simulink model "sampleModel15090_1"  (R2023b)
settings: Solver=VariableStepAuto  StartTime=0.0  StopTime=10.0  RelTol=1e-3
libraries: hdlsllib x12, simulink x2
settings Model: Creator=Tsmc  LastModifiedBy=Tsmc

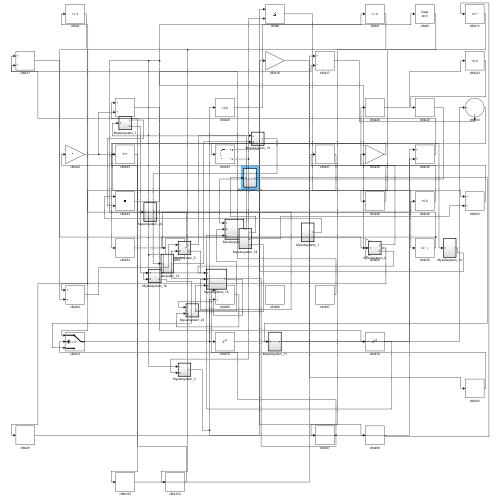
[thumbnail: Simulink's stored preview of the top-level diagram]
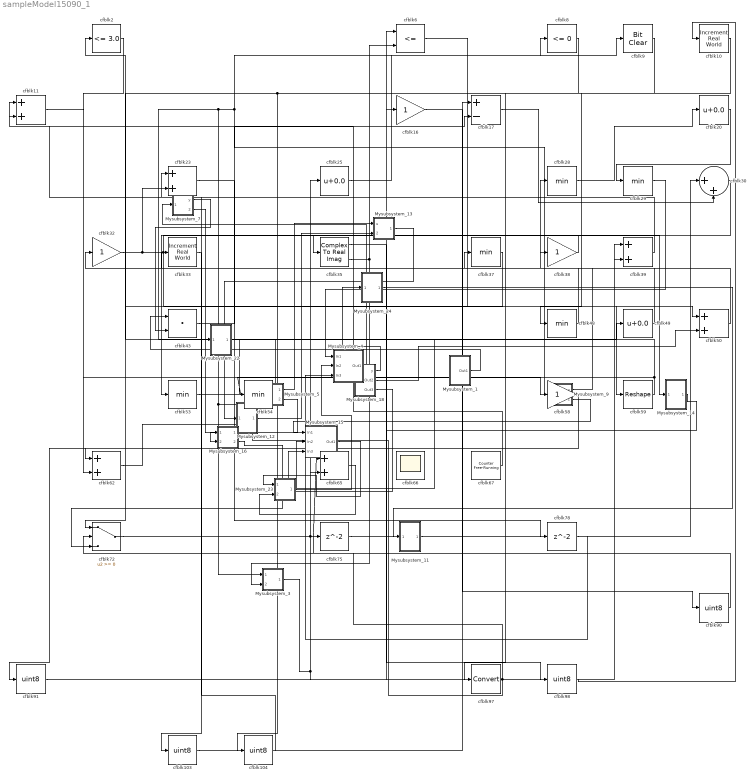
== system sampleModel15090_1 ==
  Mysubsystem_1 : Subsystem  TreatAsAtomicUnit=on  RTWFcnName=Mysubsystem_1
      settings: RTWFcnNameOpts=User specified  RTWFileNameOpts=Use function name
  Mysubsystem_11 : Subsystem  TreatAsAtomicUnit=on  RTWFcnName=Mysubsystem_11
      settings: RTWFcnNameOpts=User specified  RTWFileNameOpts=Use function name
  Mysubsystem_12 : Subsystem  TreatAsAtomicUnit=on  RTWFcnName=Mysubsystem_12
      settings: RTWFcnNameOpts=User specified  RTWFileNameOpts=Use function name
  Mysubsystem_13 : Subsystem  TreatAsAtomicUnit=on  RTWFcnName=Mysubsystem_13
      settings: RTWFcnNameOpts=User specified  RTWFileNameOpts=Use function name
  Mysubsystem_14 : Subsystem  TreatAsAtomicUnit=on  RTWFcnName=Mysubsystem_14
      settings: RTWFcnNameOpts=User specified  RTWFileNameOpts=Use function name
  Mysubsystem_15 : Subsystem  TreatAsAtomicUnit=on  RTWFcnName=Mysubsystem_15
      settings: RTWFcnNameOpts=User specified  RTWFileNameOpts=Use function name
  Mysubsystem_16 : Subsystem  TreatAsAtomicUnit=on  RTWFcnName=Mysubsystem_16
      settings: RTWFcnNameOpts=User specified  RTWFileNameOpts=Use function name
  Mysubsystem_18 : Subsystem  TreatAsAtomicUnit=on  RTWFcnName=Mysubsystem_18
      settings: RTWFcnNameOpts=User specified  RTWFileNameOpts=Use function name
  Mysubsystem_22 : Subsystem  TreatAsAtomicUnit=on  RTWFcnName=Mysubsystem_22
      settings: RTWFcnNameOpts=User specified  RTWFileNameOpts=Use function name
  Mysubsystem_23 : Subsystem  TreatAsAtomicUnit=on  RTWFcnName=Mysubsystem_23
      settings: RTWFcnNameOpts=User specified  RTWFileNameOpts=Use function name
  Mysubsystem_24 : Subsystem  TreatAsAtomicUnit=on  RTWFcnName=Mysubsystem_24
      settings: RTWFcnNameOpts=User specified  RTWFileNameOpts=Use function name
  Mysubsystem_3 : Subsystem  TreatAsAtomicUnit=on  RTWFcnName=Mysubsystem_3
      settings: RTWFcnNameOpts=User specified  RTWFileNameOpts=Use function name
  Mysubsystem_4 : Subsystem  TreatAsAtomicUnit=on  RTWFcnName=Mysubsystem_4
      settings: RTWFcnNameOpts=User specified  RTWFileNameOpts=Use function name
  Mysubsystem_5 : Subsystem  TreatAsAtomicUnit=on  RTWFcnName=Mysubsystem_5
      settings: RTWFcnNameOpts=User specified  RTWFileNameOpts=Use function name
  Mysubsystem_7 : Subsystem  TreatAsAtomicUnit=on  RTWFcnName=Mysubsystem_7
      settings: RTWFcnNameOpts=User specified  RTWFileNameOpts=Use function name
  Mysubsystem_9 : Subsystem  TreatAsAtomicUnit=on  RTWFcnName=Mysubsystem_9
      settings: RTWFcnNameOpts=User specified  RTWFileNameOpts=Use function name
  cfblk10 : hdlsllib/Math Operations/Increment Real World
  cfblk{90..91,98,103..104} (5 alike) : DataTypeConversion  OutDataTypeStr=uint8  SaturateOnIntegerOverflow=off  RndMeth=Floor
  cfblk{11,23,39,50,62,65} (6 alike) : Sum
  cfblk{16,32,38,58} (4 alike) : Gain
  cfblk17 : Sum  Inputs=+-
  cfblk2 : hdlsllib/Logic and Bit Operations/Compare To Constant  relop=<=  const=3.0  OutDataTypeStr=boolean
  cfblk20 : Bias  Bias=0.0  SaturateOnIntegerOverflow=off
  cfblk25 : Bias  Bias=0.0  SaturateOnIntegerOverflow=off
  cfblk{28..29,37,48,53..54} (6 alike) : MinMax
  cfblk30 : Sum  Inputs=|++
  cfblk33 : hdlsllib/Math Operations/Increment Real World
  cfblk35 : ComplexToRealImag
  cfblk43 : DotProduct  OutDataTypeStr=Inherit: Inherit via internal rule
  cfblk49 : Bias  Bias=0.0  SaturateOnIntegerOverflow=off
  cfblk59 : Reshape
  cfblk6 : RelationalOperator  Operator=<=  OutDataTypeStr=boolean  InputSameDT=off
  cfblk66 : Scope
      settings: Floating=on
  cfblk67 : hdlsllib/Sources/Counter Free-Running  NumBits=16  tsamp=-1
  cfblk72 : Switch  SaturateOnIntegerOverflow=off  InputSameDT=off
  cfblk75 : Delay  SampleTime=1
  cfblk78 : Delay  SampleTime=1
  cfblk8 : hdlsllib/Logic and Bit Operations/Compare To Zero  relop=<=  OutDataTypeStr=boolean
  cfblk9 : simulink/Logic and Bit Operations/Bit Clear  iBit=0
      settings: LibrarySourceBlock=|
      | hdlsllib/Logic and Bit
      | Operations/Bit Clear
  cfblk97 : DataTypeConversion  SaturateOnIntegerOverflow=off  RndMeth=Floor
  wires:
  cfblk32/1 -> Mysubsystem_14/1(In1), cfblk50/1, cfblk23/2
  cfblk72/1 -> cfblk25/1, cfblk65/1
  cfblk6/1 -> cfblk59/1
  cfblk35/2 -> Mysubsystem_3/2(In2), cfblk6/2
  cfblk20/1 -> cfblk29/1
  cfblk25/1 -> cfblk8/1
  cfblk48/1 -> cfblk2/1
  cfblk67/1 -> cfblk11/1
  cfblk28/1 -> cfblk20/1
  cfblk30/1 -> cfblk53/1
  cfblk50/1 -> cfblk28/1
  cfblk8/1 -> cfblk62/1, cfblk104/1
  cfblk10/1 -> cfblk97/1
  cfblk2/1 -> cfblk62/2
  cfblk43/1 -> cfblk17/2
  cfblk17/1 -> cfblk30/2
  cfblk53/1 -> cfblk49/1
  cfblk37/1 -> cfblk72/1
  cfblk9/1 -> cfblk48/1
  cfblk38/1 -> cfblk35/1
  cfblk49/1 -> cfblk38/1
  cfblk59/1 -> cfblk54/1, cfblk32/1
  cfblk11/1 -> cfblk58/1
  cfblk54/1 -> cfblk23/1
  cfblk39/1 -> cfblk11/2
  cfblk75/1 -> cfblk30/1
  cfblk23/1 -> cfblk78/1
  cfblk78/1 -> cfblk39/1
  cfblk16/1 -> cfblk90/1
  cfblk90/1 -> cfblk72/2
  cfblk58/1 -> cfblk91/1
  cfblk91/1 -> cfblk16/1
  cfblk97/1 -> Mysubsystem_5/2(In2), cfblk75/1
  cfblk35/1 -> cfblk98/1
  cfblk98/1 -> cfblk10/1
  cfblk33/1 -> cfblk103/1
  cfblk103/1 -> cfblk17/1
  cfblk104/1 -> cfblk33/1
  Mysubsystem_1/1(Out1) -> cfblk43/1
  Mysubsystem_3/1(Out1) -> cfblk39/2, cfblk65/2
  cfblk29/1 -> Mysubsystem_4/1(In1)
  cfblk62/1 -> Mysubsystem_5/1(In1)
  Mysubsystem_4/1(Out1) -> Mysubsystem_7/1(In1)
  Mysubsystem_7/1(y) -> cfblk43/2
  Mysubsystem_9/1(y) -> cfblk37/1
  Mysubsystem_11/1(Out1) -> Mysubsystem_4/3(In3)
  Mysubsystem_5/1(Out1) -> Mysubsystem_13/1(u)
  Mysubsystem_12/1(Out1) -> Mysubsystem_13/2(In2)
  Mysubsystem_13/1(Out1) -> Mysubsystem_12/1(In1)
  Mysubsystem_14/1(Out1) -> cfblk6/1
  Mysubsystem_9/2(Out2) -> Mysubsystem_15/1(In1)
  Mysubsystem_16/1(Out1) -> Mysubsystem_9/1(In1), cfblk9/1, Mysubsystem_22/1(In1), Mysubsystem_3/1(In1)
  Mysubsystem_7/2(Out2) -> Mysubsystem_16/1(In1)
  Mysubsystem_5/2(Out2) -> Mysubsystem_16/2(In2)
  Mysubsystem_16/2(Out2) -> cfblk72/3
  Mysubsystem_18/2(Out2) -> cfblk50/2
  Mysubsystem_18/3(Out3) -> Mysubsystem_15/3(In3)
  Mysubsystem_22/1(Out1) -> Mysubsystem_15/2(In2)
  Mysubsystem_15/1(Out1) -> Mysubsystem_23/1(In1)
  cfblk65/1 -> Mysubsystem_23/2(In2)
  Mysubsystem_23/1(Out1) -> Mysubsystem_4/2(In2)
  Mysubsystem_18/1(y) -> Mysubsystem_24/1(In1)
  Mysubsystem_24/1(Out1) -> Mysubsystem_11/1(In1)

== system sampleModel15090_1/Mysubsystem_1 ==
  cfblk34 : hdlsllib/Math Operations/Increment Real World
  cfblk46 : Abs  SaturateOnIntegerOverflow=off
  cfblk80 : Delay  SampleTime=1
  Out1 : Outport
  wires:
  cfblk46/1 -> Out1/1, cfblk80/1
  cfblk34/1 -> cfblk46/1
  cfblk80/1 -> cfblk34/1

== system sampleModel15090_1/Mysubsystem_11 ==
  In1 : Inport
  cfblk51 : Reshape
  cfblk88 : DataTypeConversion  OutDataTypeStr=uint8  SaturateOnIntegerOverflow=off  RndMeth=Floor
  cfblk89 : DataTypeConversion  OutDataTypeStr=uint8  SaturateOnIntegerOverflow=off  RndMeth=Floor
  Out1 : Outport
  wires:
  cfblk88/1 -> Out1/1
  cfblk51/1 -> cfblk88/1
  cfblk89/1 -> cfblk51/1
  In1/1 -> cfblk89/1

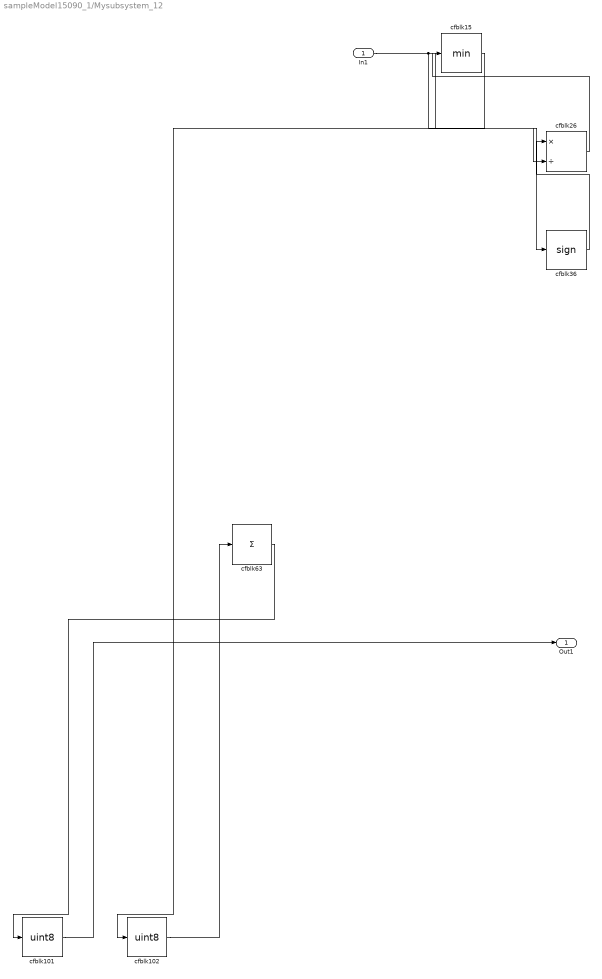
== system sampleModel15090_1/Mysubsystem_12 ==
  In1 : Inport
  cfblk101 : DataTypeConversion  OutDataTypeStr=uint8  SaturateOnIntegerOverflow=off  RndMeth=Floor
  cfblk102 : DataTypeConversion  OutDataTypeStr=uint8  SaturateOnIntegerOverflow=off  RndMeth=Floor
  cfblk15 : MinMax
  cfblk26 : Product  Inputs=*/  RndMeth=Zero  SaturateOnIntegerOverflow=on
  cfblk36 : Signum
  cfblk63 : Sum  Inputs=+
  Out1 : Outport
  wires:
  cfblk36/1 -> cfblk26/1
  cfblk101/1 -> Out1/1
  cfblk26/1 -> cfblk15/1
  In1/1 -> cfblk36/1, cfblk26/2
  cfblk63/1 -> cfblk101/1
  cfblk102/1 -> cfblk63/1
  cfblk15/1 -> cfblk102/1

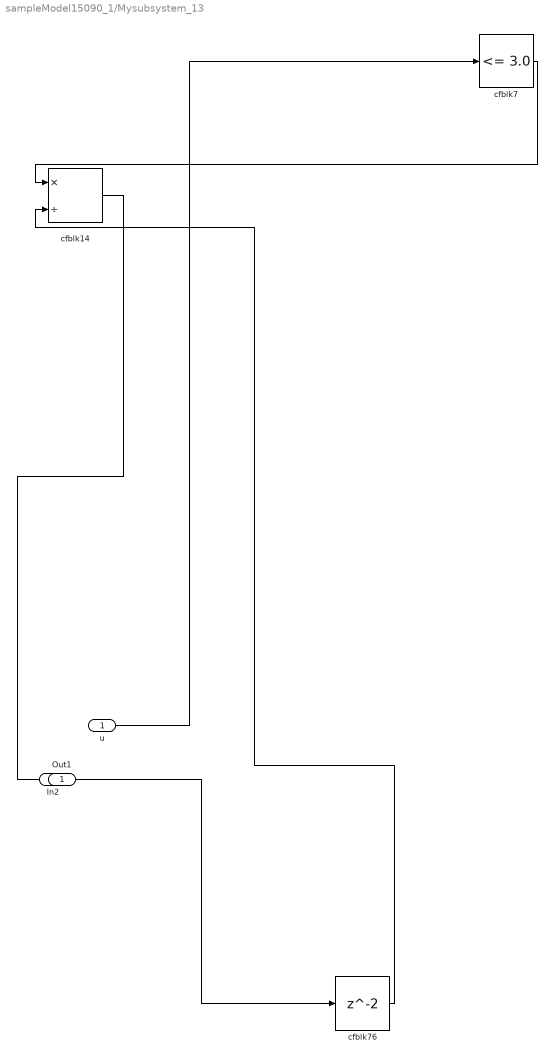
== system sampleModel15090_1/Mysubsystem_13 ==
  u : Inport
  In2 : Inport  Port=2
  cfblk14 : Product  Inputs=*/  RndMeth=Zero  SaturateOnIntegerOverflow=on
  cfblk7 : hdlsllib/Logic and Bit Operations/Compare To Constant  relop=<=  const=3.0  OutDataTypeStr=boolean
  cfblk76 : Delay  SampleTime=1
  Out1 : Outport
  wires:
  cfblk7/1 -> cfblk14/1
  In2/1 -> cfblk76/1
  cfblk14/1 -> Out1/1
  cfblk76/1 -> cfblk14/2
  u/1 -> cfblk7/1

== system sampleModel15090_1/Mysubsystem_14 ==
  In1 : Inport
  cfblk40 : Abs  SaturateOnIntegerOverflow=off
  cfblk79 : Delay  SampleTime=1
  Out1 : Outport
  wires:
  cfblk40/1 -> cfblk79/1
  In1/1 -> cfblk40/1
  cfblk79/1 -> Out1/1

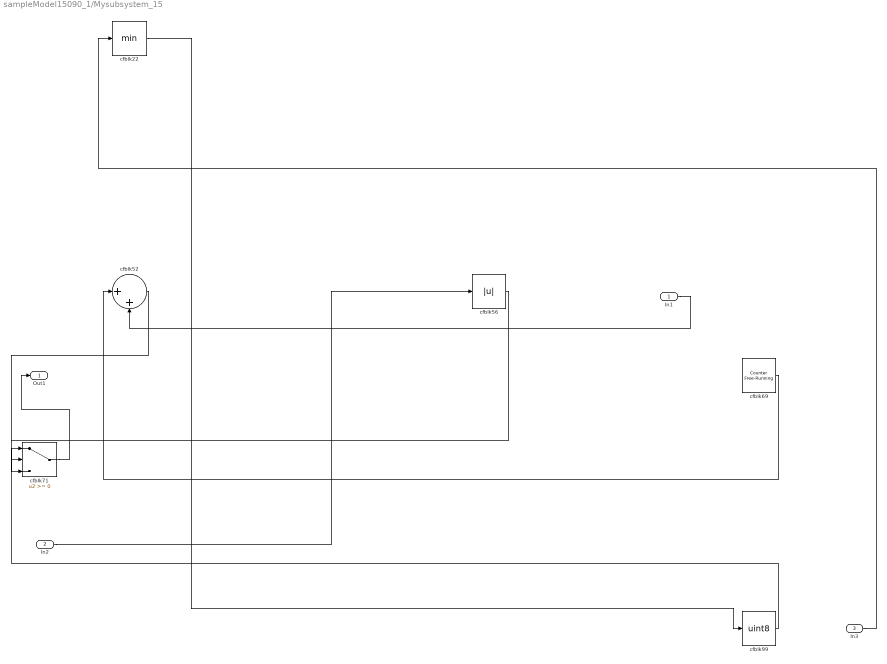
== system sampleModel15090_1/Mysubsystem_15 ==
  In1 : Inport
  In2 : Inport  Port=2
  In3 : Inport  Port=3
  cfblk22 : MinMax
  cfblk52 : Sum  Inputs=|++
  cfblk56 : Abs  SaturateOnIntegerOverflow=off
  cfblk69 : hdlsllib/Sources/Counter Free-Running  NumBits=16  tsamp=-1
  cfblk71 : Switch  SaturateOnIntegerOverflow=off  InputSameDT=off
  cfblk99 : DataTypeConversion  OutDataTypeStr=uint8  SaturateOnIntegerOverflow=off  RndMeth=Floor
  Out1 : Outport
  wires:
  cfblk69/1 -> cfblk52/1
  cfblk52/1 -> cfblk71/2
  cfblk22/1 -> cfblk99/1
  cfblk99/1 -> cfblk71/1
  cfblk56/1 -> cfblk71/3
  cfblk71/1 -> Out1/1
  In2/1 -> cfblk56/1
  In3/1 -> cfblk22/1
  In1/1 -> cfblk52/2

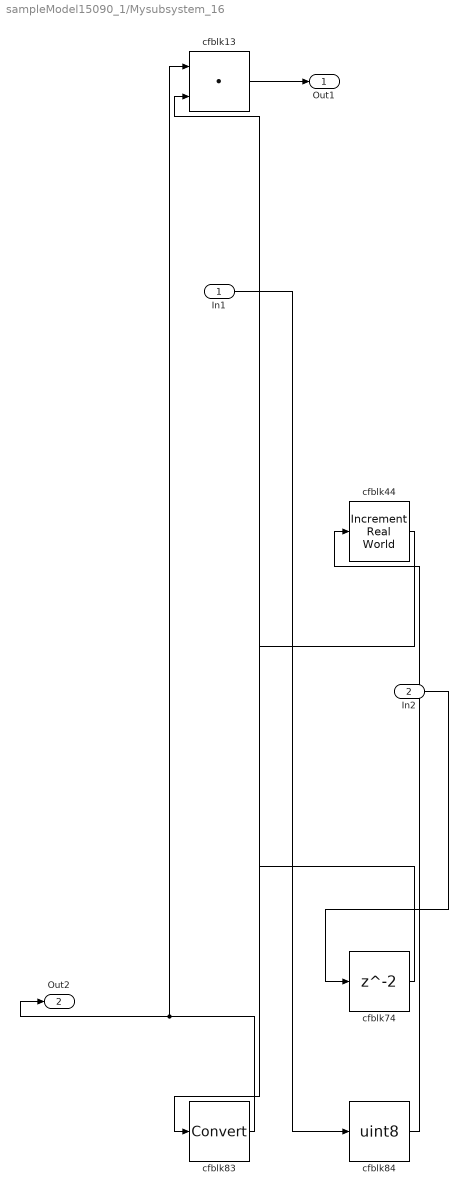
== system sampleModel15090_1/Mysubsystem_16 ==
  In1 : Inport
  In2 : Inport  Port=2
  cfblk13 : DotProduct  OutDataTypeStr=Inherit: Inherit via internal rule
  cfblk44 : hdlsllib/Math Operations/Increment Real World
  cfblk74 : Delay  SampleTime=1
  cfblk83 : DataTypeConversion  SaturateOnIntegerOverflow=off  RndMeth=Floor
  cfblk84 : DataTypeConversion  OutDataTypeStr=uint8  SaturateOnIntegerOverflow=off  RndMeth=Floor
  Out1 : Outport
  Out2 : Outport  Port=2
  wires:
  cfblk44/1 -> cfblk83/1
  cfblk84/1 -> cfblk44/1
  In2/1 -> cfblk74/1
  cfblk13/1 -> Out1/1
  cfblk74/1 -> cfblk13/2
  cfblk83/1 -> Out2/1, cfblk13/1
  In1/1 -> cfblk84/1

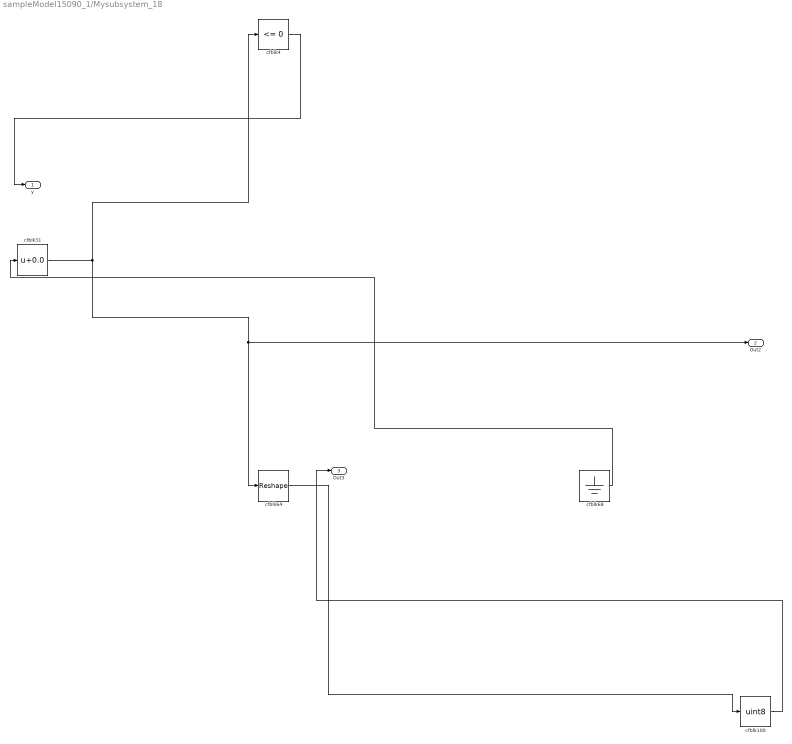
== system sampleModel15090_1/Mysubsystem_18 ==
  cfblk100 : DataTypeConversion  OutDataTypeStr=uint8  SaturateOnIntegerOverflow=off  RndMeth=Floor
  cfblk31 : Bias  Bias=0.0  SaturateOnIntegerOverflow=off
  cfblk4 : hdlsllib/Logic and Bit Operations/Compare To Zero  relop=<=  OutDataTypeStr=boolean
  cfblk64 : Reshape
  cfblk68 : Ground
  y : Outport
  Out2 : Outport  Port=2
  Out3 : Outport  Port=3
  wires:
  cfblk31/1 -> Out2/1, cfblk64/1, cfblk4/1
  cfblk64/1 -> cfblk100/1
  cfblk68/1 -> cfblk31/1
  cfblk4/1 -> y/1
  cfblk100/1 -> Out3/1

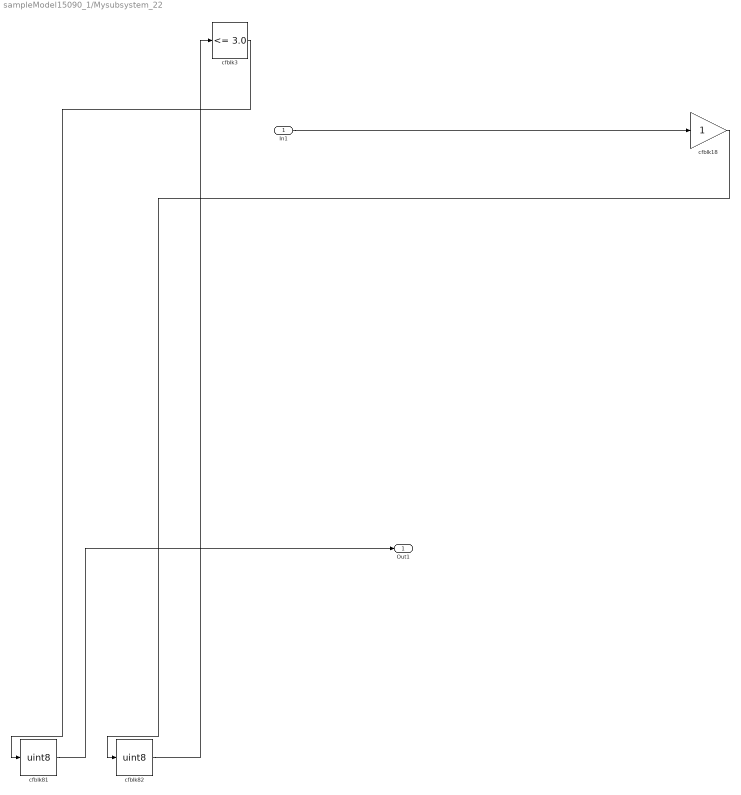
== system sampleModel15090_1/Mysubsystem_22 ==
  In1 : Inport
  cfblk18 : Gain
  cfblk3 : hdlsllib/Logic and Bit Operations/Compare To Constant  relop=<=  const=3.0  OutDataTypeStr=boolean
  cfblk81 : DataTypeConversion  OutDataTypeStr=uint8  SaturateOnIntegerOverflow=off  RndMeth=Floor
  cfblk82 : DataTypeConversion  OutDataTypeStr=uint8  SaturateOnIntegerOverflow=off  RndMeth=Floor
  Out1 : Outport
  wires:
  cfblk18/1 -> cfblk82/1
  In1/1 -> cfblk18/1
  cfblk82/1 -> cfblk3/1
  cfblk3/1 -> cfblk81/1
  cfblk81/1 -> Out1/1

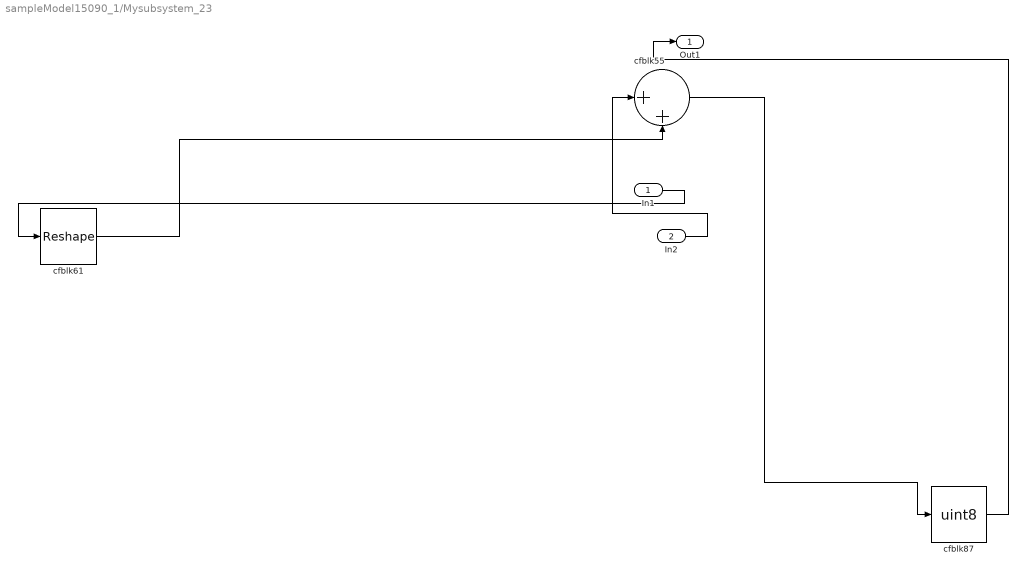
== system sampleModel15090_1/Mysubsystem_23 ==
  In1 : Inport
  In2 : Inport  Port=2
  cfblk55 : Sum  Inputs=|++
  cfblk61 : Reshape
  cfblk87 : DataTypeConversion  OutDataTypeStr=uint8  SaturateOnIntegerOverflow=off  RndMeth=Floor
  Out1 : Outport
  wires:
  cfblk55/1 -> cfblk87/1
  cfblk61/1 -> cfblk55/2
  In2/1 -> cfblk55/1
  In1/1 -> cfblk61/1
  cfblk87/1 -> Out1/1

== system sampleModel15090_1/Mysubsystem_24 ==
  In1 : Inport
  cfblk21 : Signum
  cfblk60 : Reshape
  Out1 : Outport
  wires:
  cfblk21/1 -> cfblk60/1
  In1/1 -> cfblk21/1
  cfblk60/1 -> Out1/1

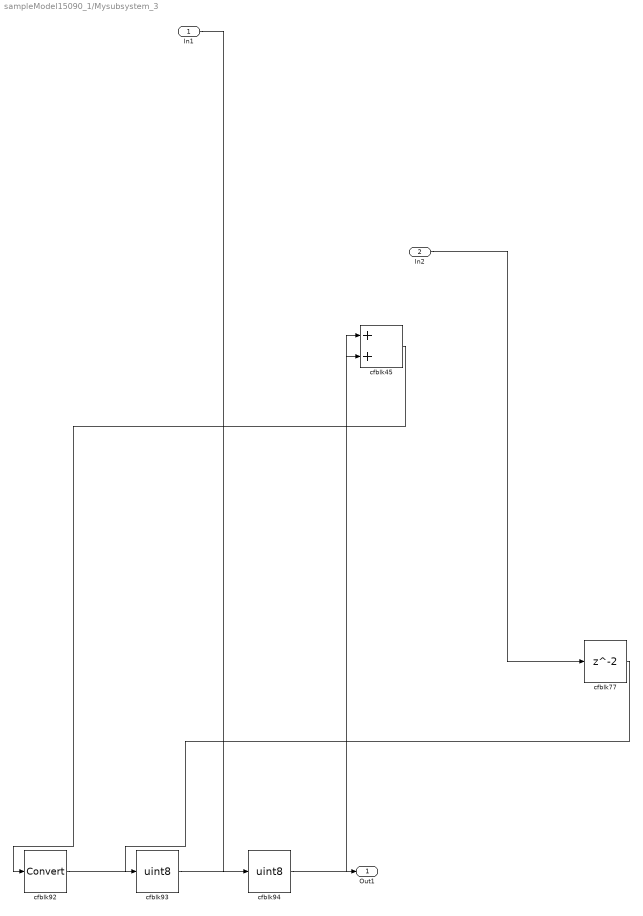
== system sampleModel15090_1/Mysubsystem_3 ==
  In1 : Inport
  In2 : Inport  Port=2
  cfblk45 : Sum
  cfblk77 : Delay  SampleTime=1
  cfblk92 : DataTypeConversion  SaturateOnIntegerOverflow=off  RndMeth=Floor
  cfblk93 : DataTypeConversion  OutDataTypeStr=uint8  SaturateOnIntegerOverflow=off  RndMeth=Floor
  cfblk94 : DataTypeConversion  OutDataTypeStr=uint8  SaturateOnIntegerOverflow=off  RndMeth=Floor
  Out1 : Outport
  wires:
  In2/1 -> cfblk77/1
  cfblk45/1 -> cfblk92/1
  cfblk92/1 -> Out1/1
  In1/1 -> cfblk94/1
  cfblk77/1 -> cfblk93/1
  cfblk94/1 -> cfblk45/2
  cfblk93/1 -> cfblk45/1

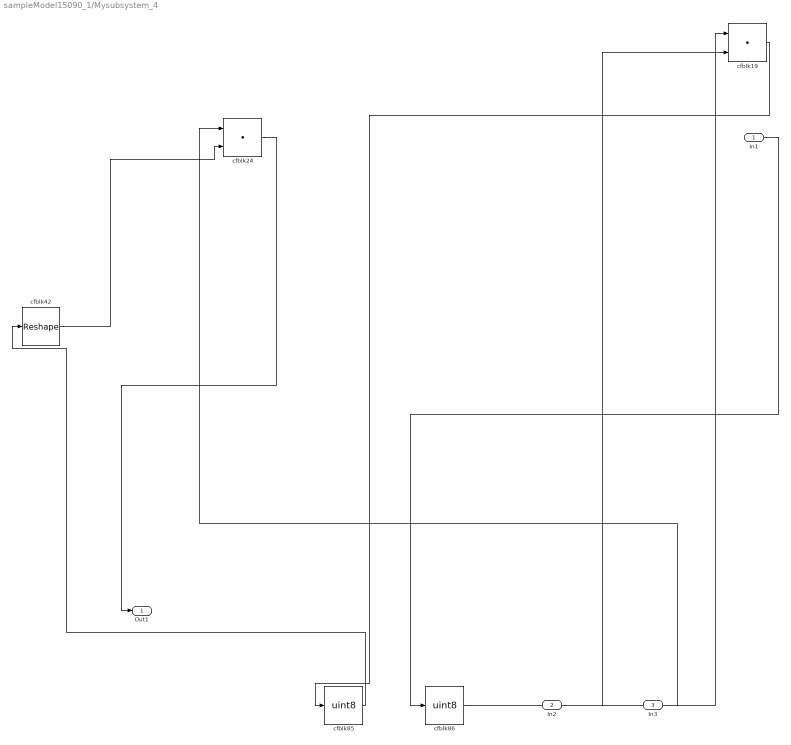
== system sampleModel15090_1/Mysubsystem_4 ==
  In1 : Inport
  In2 : Inport  Port=2
  In3 : Inport  Port=3
  cfblk19 : DotProduct  OutDataTypeStr=Inherit: Inherit via internal rule
  cfblk24 : DotProduct  OutDataTypeStr=Inherit: Inherit via internal rule
  cfblk42 : Reshape
  cfblk85 : DataTypeConversion  OutDataTypeStr=uint8  SaturateOnIntegerOverflow=off  RndMeth=Floor
  cfblk86 : DataTypeConversion  OutDataTypeStr=uint8  SaturateOnIntegerOverflow=off  RndMeth=Floor
  Out1 : Outport
  wires:
  cfblk24/1 -> Out1/1
  In1/1 -> cfblk86/1
  cfblk42/1 -> cfblk24/2
  cfblk19/1 -> cfblk85/1
  cfblk86/1 -> cfblk19/1
  In3/1 -> cfblk24/1
  cfblk85/1 -> cfblk42/1
  In2/1 -> cfblk19/2

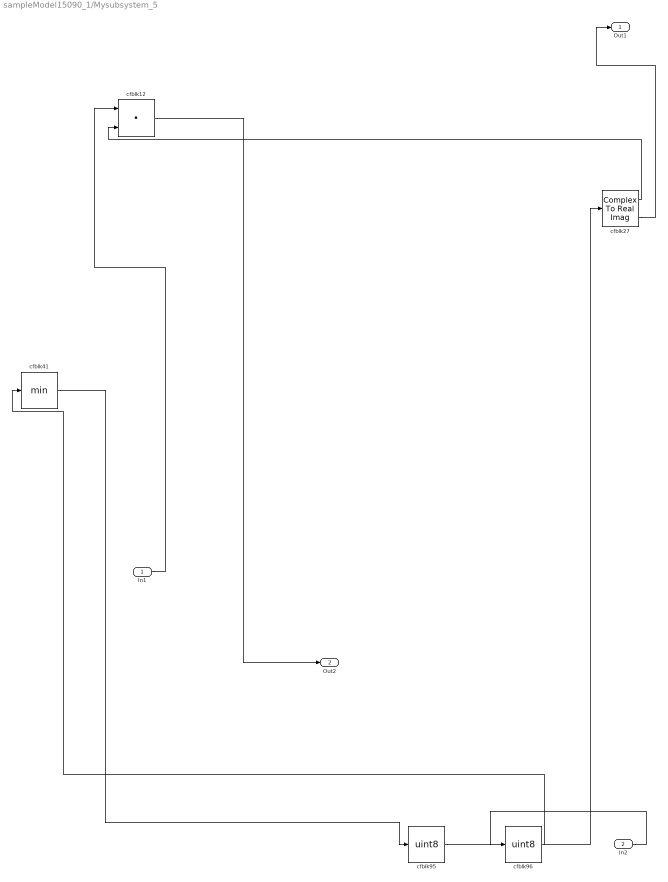
== system sampleModel15090_1/Mysubsystem_5 ==
  In1 : Inport
  In2 : Inport  Port=2
  cfblk12 : DotProduct  OutDataTypeStr=Inherit: Inherit via internal rule
  cfblk27 : ComplexToRealImag
  cfblk41 : MinMax
  cfblk95 : DataTypeConversion  OutDataTypeStr=uint8  SaturateOnIntegerOverflow=off  RndMeth=Floor
  cfblk96 : DataTypeConversion  OutDataTypeStr=uint8  SaturateOnIntegerOverflow=off  RndMeth=Floor
  Out1 : Outport
  Out2 : Outport  Port=2
  wires:
  cfblk27/2 -> Out1/1
  cfblk41/1 -> cfblk95/1
  cfblk96/1 -> cfblk41/1
  cfblk95/1 -> cfblk27/1
  cfblk12/1 -> Out2/1
  cfblk27/1 -> cfblk12/2
  In2/1 -> cfblk96/1
  In1/1 -> cfblk12/1

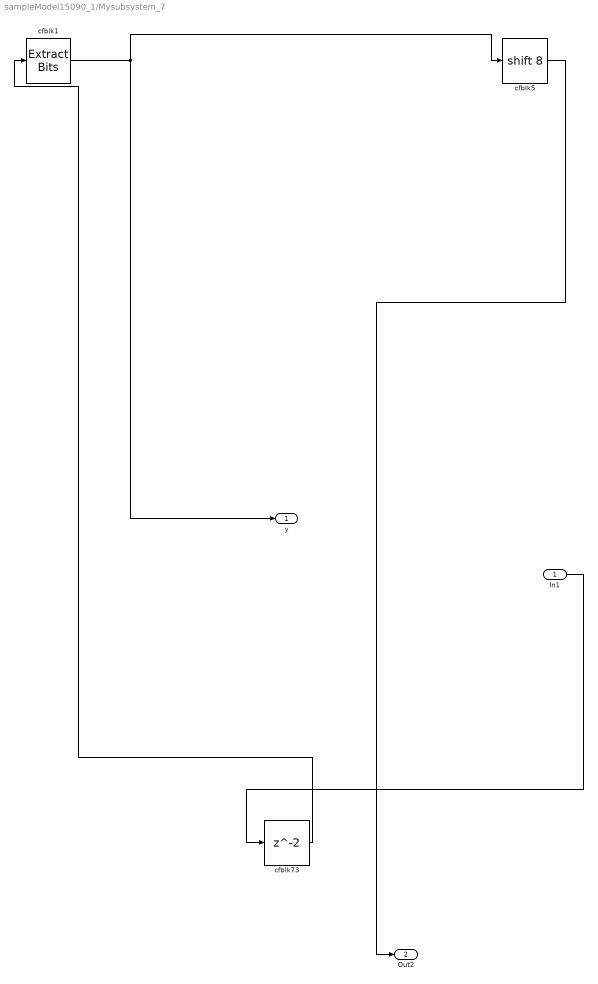
== system sampleModel15090_1/Mysubsystem_7 ==
  In1 : Inport
  cfblk1 : simulink/Logic and Bit Operations/Extract Bits  bitsToExtract=Upper half  numBits=8  bitIdxRange=[0 7]  outScalingMode=Preserve fixed-point scaling
      settings: LibrarySourceBlock=|
      | hdlsllib/Logic and Bit
      | Operations/Extract Bits
  cfblk5 : ArithShift  BitShiftNumber=8
  cfblk73 : Delay  SampleTime=1
  y : Outport
  Out2 : Outport  Port=2
  wires:
  In1/1 -> cfblk73/1
  cfblk73/1 -> cfblk1/1
  cfblk1/1 -> y/1, cfblk5/1
  cfblk5/1 -> Out2/1

== system sampleModel15090_1/Mysubsystem_9 ==
  In1 : Inport
  cfblk47 : Reshape
  cfblk57 : Sum  Inputs=+-
  cfblk70 : hdlsllib/Sources/Counter Limited  uplimit=7  tsamp=-1
  y : Outport
  Out2 : Outport  Port=2
  wires:
  cfblk57/1 -> cfblk47/1
  In1/1 -> cfblk57/2
  cfblk70/1 -> y/1, cfblk57/1
  cfblk47/1 -> Out2/1
